simulink model "MSDRPrimaryLoop_LoadFollow"  (R2021b)
settings: Solver=VariableStepAuto  StartTime=0.0  StopTime=604900  MaxStep=1  MinStep=0.01  RelTol=1e-3
undefined symbols (not defined in the file): a_f, A_free_PHX, a_g, A_h_PHX, beta, beta_t, bubbleGeneratorArea, bubbleGeneratorDh, bubbleGeneratorElevation, bubbleGeneratorLength, bubbleGeneratorVolume, bubbleSaturationLevel, bubbleSeparatorArea, bubbleSeparatorDiameter, bubbleSeparatorDo, bubbleSeparatorLength, bubbleSeparatorSlope, bypassRatio, C0, coreFlowArea, coreFuelVolume, coreLowerPlenumArea, coreLowerPlenumHydraulicDiameter, coreLowerPlenumLength, coreLowerPlenumVolume, coreUpperPlenumArea, coreUpperPlenumHydraulicDiameter, coreUpperPlenumLength, coreUpperPlenumVolume, coreVolume, cpGraphite, dissolusionRatio, dMin, dScale, dsmConst, DXeG, Fiss_factor, fuelChannelHydrualicDiameter, fuelChannelLength, fuelDepositRatio, fuelFraction, fuelGraphiteArea, fuelGraphiteHeatTransferCoefficient, gamma0, gamma1, gamma2, generatorDsm, graphiteKDiff, graphiteUnitCellThickness, initialIodineConcentration, InitialXeMolarConcentration, InjectionRatio, injectionRatio, iodineDecayConstant, IodineDecayConstant, iodineYield, kGraphite, kScale, Lam, lam ... (+60)
libraries: fl_lib x268, nesl_utility x106, SimscapeFluids_lib x20, slpidlib x1
(part 7 of 12)

== system MSDRPrimaryLoop_LoadFollow/pipeReactorToPump/XenonCalc/Gas ==
  XeGIn : Inport
  Interphase : Inport  Port=2
  GasRef : Inport  Port=3
  VolumeRate : Inport  Port=4
  Add : Sum  Inputs=+---
  Add1 : Sum  Inputs=+-
  Add2 : Sum
  Constant : Constant
  Gain2 : Gain  Gain=xeDecayConstant
  Gain4 : Gain  Gain=0.5/Area
  LiquidFlowRate : Product
  LiquidVolume : Product  Inputs=*/
  MixtureVolume : Gain  Gain=1/Volume
  PhaseMass : Integrator  LimitOutput=on  LowerSaturationLimit=0
  Subsystem : Subsystem  ReferencedSubsystem=GasToAlpha
  XeGOut : Outport
  GxGas : Outport  Port=2
  wires:
  LiquidFlowRate/1 -> XeGOut/1, Add2/2, Add/3
  Subsystem/1 -> Add1/2
  LiquidVolume/1 -> LiquidFlowRate/2
  Add/1 -> PhaseMass/1
  Constant/1 -> Add1/1
  MixtureVolume/1 -> LiquidVolume/1
  Add1/1 -> LiquidVolume/2
  VolumeRate/1 -> LiquidFlowRate/1
  GasRef/1 -> Subsystem/1
  XeGIn/1 -> Add/1, Add2/1
  Gain2/1 -> Add/4
  PhaseMass/1 -> Gain2/1, MixtureVolume/1
  Gain4/1 -> GxGas/1
  Add2/1 -> Gain4/1
  Interphase/1 -> Add/2

== system MSDRPrimaryLoop_LoadFollow/pipeReactorToPump/XenonCalc/InterphaseTranfser ==
  note: This local to volume isn't strick. Either add an integral or reduce the length of the node if variation is large.
  GxSalt : Inport
  GasRef : Inport  Port=2
  GxGas : Inport  Port=3
  PLoss : Inport  Port=4
  VolumeRate : Inport  Port=5
  Constant : Constant  Value=Dh
  Constitutive : Subsystem
      settings: PortSchema="{\"entries\":[{\"content\":{\"sides\":[{\"content\":{\"connectorIds\":[\"In1\",\"LConn1\",\"In2\",\"In3\",\"In4\"]},\"type\":\"ConnectorPlacement.EquallySpacedRectSide\",\"uuid\":\"b30af6c3-7c55-4661-bc76-939f1c8a4177\"},{\"content\":{\"connectorIds\":[\"Out1\",\"Out2\",\"Out3\",\"Out4\",\"Out5\",\"Out6\",\"Out7\",\"Out8\",\"Out9\"],\"side\":\"RIGHT\"},\"type\":\"ConnectorPlacement.EquallySpacedRectSide\",\"uuid\":\"0b137634-5e01-4bd6-8381-72b0699f5835\"},{\"content\":{\"connectorIds\":[],\"side\":\"TOP\"},\"type\":\"ConnectorPlacement.EquallySpacedRectSide\",\"uuid\":\"06046061-3240-493e-a0a3-282c9541adae\"}]},\"type\":\"ConnectorPlacement.EquallySpacedConnector\",\"uuid\":\"b0591291-fd4b-4355-beaa-e569a19c4b12\"}],\"packageUris\":[\"http://schema.mathworks.com/mf0/Connector/R2020b\"],\"version\":\"1.0\"}"
  MixtureVolume : Gain  Gain=Volume
  String Constant : StringConstant  String="\"upwards\""
  Subsystem : Subsystem  ReferencedSubsystem=kCalculation
      settings: PortSchema="{\"entries\":[{\"content\":{\"sides\":[{\"content\":{\"connectorIds\":[\"In2\",\"In3\",\"In4\",\"In5\",\"In6\",\"In7\",\"In8\",\"In1\"]},\"type\":\"ConnectorPlacement.EquallySpacedRectSide\",\"uuid\":\"002a6616-4b3b-4d3e-9efd-a784f6bbe134\"},{\"content\":{\"connectorIds\":[\"Out1\",\"Out2\"],\"side\":\"RIGHT\"},\"type\":\"ConnectorPlacement.EquallySpacedRectSide\",\"uuid\":\"da6acc14-6515-461b-8149-f4cbf493a4dd\"},{\"content\":{\"connectorIds\":[],\"side\":\"TOP\"},\"type\":\"ConnectorPlacement.EquallySpacedRectSide\",\"uuid\":\"939e49a4-f3cd-4ed3-a7a5-6bbefe0ae08a\"}]},\"type\":\"ConnectorPlacement.EquallySpacedConnector\",\"uuid\":\"8f0c794e-eb76-47c6-abaf-8e07cad1f307\"}],\"packageUris\":[\"http://schema.mathworks.com/mf0/Connector/R2020b\"],\"version\":\"1.0\"}"
  Subsystem1 : Subsystem  ReferencedSubsystem=GasToAlpha
  Transfer Term : MATLAB Function  TreatAsAtomicUnit=on
  Ref : PMIOPort  Side=Left
  TranfserRate : Outport
  wires:
  Transfer Term/1(volRate) -> MixtureVolume/1
  MixtureVolume/1 -> TranfserRate/1
  VolumeRate/1 -> Constitutive/3(VolumeRate)
  GasRef/1 -> Subsystem1/1
  Subsystem1/1 -> Constitutive/1(alpha), Transfer Term/3(alpha)
  Constitutive/1(ul) -> Transfer Term/4(ul)
  Constitutive/2(ug) -> Transfer Term/5(ug)
  Constant/1 -> Subsystem/7, Constitutive/4(Diam)
  GxSalt/1 -> Transfer Term/1(GxS)
  GxGas/1 -> Transfer Term/2(GxG)
  Subsystem/1 -> Transfer Term/7(dsm)
  Subsystem/2 -> Transfer Term/8(k)
  PLoss/1 -> Constitutive/2(PLoss)
  Constitutive/4(Re) -> Subsystem/2
  Constitutive/3(K) -> Transfer Term/6(K)
  Constitutive/5(Sc) -> Subsystem/3
  Constitutive/6(Diff) -> Subsystem/4
  Constitutive/7(alphaC) -> Subsystem/5
  Constitutive/8(dsm) -> Subsystem/6
  Constitutive/9(f_m) -> Subsystem/1
  String Constant/1 -> Subsystem/8
  connections:
  Constitutive/LConn1 -- Ref/RConn1

== system MSDRPrimaryLoop_LoadFollow/pipeReactorToPump/XenonCalc/Salt ==
  XeLIn : Inport  PortDimensions=1
  IodineSNumberDensity : Inport  Port=2  PortDimensions=1
  T_f_ave : Inport  Port=3
  GasRef : Inport  Port=4  PortDimensions=1
  VolumeRate : Inport  Port=5
  Interphase : Inport  Port=6
  Add : Sum  Inputs=+++--  InputSameDT=on
  Add1 : Sum
  Decay : Gain  Gain=xeDecayConstant
  Gain1 : Gain  Gain=0.5/Area
  InPipeGeneration : Subsystem
      settings: PortSchema="{\"entries\":[{\"content\":{\"sides\":[{\"content\":{\"connectorIds\":[\"In1\"]},\"type\":\"ConnectorPlacement.EquallySpacedRectSide\",\"uuid\":\"cf58f9e2-4051-4ec0-bfd5-a375f3464f67\"},{\"content\":{\"connectorIds\":[\"Out1\"],\"side\":\"RIGHT\"},\"type\":\"ConnectorPlacement.EquallySpacedRectSide\",\"uuid\":\"cf475b22-0422-4ebc-b148-ab559744c6ba\"},{\"content\":{\"connectorIds\":[],\"side\":\"TOP\"},\"type\":\"ConnectorPlacement.EquallySpacedRectSide\",\"uuid\":\"15cc78ce-ee79-4f49-b098-b77c0b2a8ba1\"},{\"content\":{\"connectorIds\":[\"In2\"],\"side\":\"BOTTOM\"},\"type\":\"ConnectorPlacement.EquallySpacedRectSide\",\"uuid\":\"64f5be1f-19d6-4b5f-ac24-c41659a6a539\"}]},\"type\":\"ConnectorPlacement.EquallySpacedConnector\",\"uuid\":\"1fb1607a-ceed-4d70-a511-7b706be0d7ea\"}],\"packageUris\":[\"http://schema.mathworks.com/mf0/Connector/R2020b\"],\"version\":\"1.0\"}"
  LiquidFlowRate : Product
  LiquidVolume : Product  Inputs=*/
  MixtureVolume : Gain  Gain=1/Volume
  PhaseMass : Integrator  LimitOutput=on  LowerSaturationLimit=0
  Subsystem1 : Subsystem
  XeLOut : Outport  PortDimensions=1
  GxSalt : Outport  Port=2
  wires:
  LiquidFlowRate/1 -> Add/5, XeLOut/1, Add1/2
  IodineSNumberDensity/1 -> InPipeGeneration/1(IodineSNumberDensity)
  LiquidVolume/1 -> LiquidFlowRate/2
  Add/1 -> PhaseMass/1
  MixtureVolume/1 -> LiquidVolume/1
  VolumeRate/1 -> LiquidFlowRate/1
  T_f_ave/1 -> InPipeGeneration/2(T_f_ave)
  PhaseMass/1 -> Decay/1, MixtureVolume/1
  GasRef/1 -> Subsystem1/1(Gas)
  Subsystem1/1(1-alpha) -> LiquidVolume/2
  InPipeGeneration/1("XenonGenerationRate, [kg/s]") -> Add/2
  XeLIn/1 -> Add1/1, Add/1
  Add1/1 -> Gain1/1
  Gain1/1 -> GxSalt/1
  Interphase/1 -> Add/3
  Decay/1 -> Add/4

== system MSDRPrimaryLoop_LoadFollow/Chemical Processing/Bubble Generator/XenonCalc/Gas ==
  XeGIn : Inport
  Interphase : Inport  Port=2
  GasRef : Inport  Port=3
  VolumeRate : Inport  Port=4
  Add : Sum  Inputs=+---
  Add1 : Sum  Inputs=+-
  Add2 : Sum
  Constant : Constant
  Gain2 : Gain  Gain=xeDecayConstant
  Gain4 : Gain  Gain=0.5/Area
  LiquidFlowRate : Product
  LiquidVolume : Product  Inputs=*/
  MixtureVolume : Gain  Gain=1/Volume
  PhaseMass : Integrator  LimitOutput=on  LowerSaturationLimit=0
  Subsystem : Subsystem  ReferencedSubsystem=GasToAlpha
  XeGOut : Outport
  GxGas : Outport  Port=2
  wires:
  LiquidFlowRate/1 -> XeGOut/1, Add2/2, Add/3
  Subsystem/1 -> Add1/2
  LiquidVolume/1 -> LiquidFlowRate/2
  Add/1 -> PhaseMass/1
  Constant/1 -> Add1/1
  MixtureVolume/1 -> LiquidVolume/1
  Add1/1 -> LiquidVolume/2
  VolumeRate/1 -> LiquidFlowRate/1
  GasRef/1 -> Subsystem/1
  XeGIn/1 -> Add/1, Add2/1
  Gain2/1 -> Add/4
  PhaseMass/1 -> Gain2/1, MixtureVolume/1
  Gain4/1 -> GxGas/1
  Add2/1 -> Gain4/1
  Interphase/1 -> Add/2

== system MSDRPrimaryLoop_LoadFollow/Chemical Processing/Bubble Generator/XenonCalc/InterphaseTranfser ==
  note: This local to volume isn't strick. Either add an integral or reduce the length of the node if variation is large.
  GxSalt : Inport
  GasRef : Inport  Port=2
  GxGas : Inport  Port=3
  PLoss : Inport  Port=4
  VolumeRate : Inport  Port=5
  Constant : Constant  Value=Dh
  Constitutive : Subsystem
      settings: PortSchema="{\"entries\":[{\"content\":{\"sides\":[{\"content\":{\"connectorIds\":[\"In1\",\"LConn1\",\"In2\",\"In3\",\"In4\"]},\"type\":\"ConnectorPlacement.EquallySpacedRectSide\",\"uuid\":\"b30af6c3-7c55-4661-bc76-939f1c8a4177\"},{\"content\":{\"connectorIds\":[\"Out1\",\"Out2\",\"Out3\",\"Out4\",\"Out5\",\"Out6\",\"Out7\",\"Out8\",\"Out9\"],\"side\":\"RIGHT\"},\"type\":\"ConnectorPlacement.EquallySpacedRectSide\",\"uuid\":\"0b137634-5e01-4bd6-8381-72b0699f5835\"},{\"content\":{\"connectorIds\":[],\"side\":\"TOP\"},\"type\":\"ConnectorPlacement.EquallySpacedRectSide\",\"uuid\":\"06046061-3240-493e-a0a3-282c9541adae\"}]},\"type\":\"ConnectorPlacement.EquallySpacedConnector\",\"uuid\":\"b0591291-fd4b-4355-beaa-e569a19c4b12\"}],\"packageUris\":[\"http://schema.mathworks.com/mf0/Connector/R2020b\"],\"version\":\"1.0\"}"
  MixtureVolume : Gain  Gain=Volume
  Subsystem : Subsystem  ReferencedSubsystem=kCalculation
      settings: PortSchema="{\"entries\":[{\"content\":{\"sides\":[{\"content\":{\"connectorIds\":[\"In2\",\"In3\",\"In4\",\"In5\",\"In6\",\"In7\",\"In8\",\"In1\"]},\"type\":\"ConnectorPlacement.EquallySpacedRectSide\",\"uuid\":\"002a6616-4b3b-4d3e-9efd-a784f6bbe134\"},{\"content\":{\"connectorIds\":[\"Out1\",\"Out2\"],\"side\":\"RIGHT\"},\"type\":\"ConnectorPlacement.EquallySpacedRectSide\",\"uuid\":\"da6acc14-6515-461b-8149-f4cbf493a4dd\"},{\"content\":{\"connectorIds\":[],\"side\":\"TOP\"},\"type\":\"ConnectorPlacement.EquallySpacedRectSide\",\"uuid\":\"939e49a4-f3cd-4ed3-a7a5-6bbefe0ae08a\"}]},\"type\":\"ConnectorPlacement.EquallySpacedConnector\",\"uuid\":\"8f0c794e-eb76-47c6-abaf-8e07cad1f307\"}],\"packageUris\":[\"http://schema.mathworks.com/mf0/Connector/R2020b\"],\"version\":\"1.0\"}"
  Subsystem1 : Subsystem  ReferencedSubsystem=GasToAlpha
  Transfer Term : MATLAB Function  TreatAsAtomicUnit=on
  Ref : PMIOPort  Side=Left
  TranfserRate : Outport
  wires:
  Transfer Term/1(volRate) -> MixtureVolume/1
  MixtureVolume/1 -> TranfserRate/1
  VolumeRate/1 -> Constitutive/3(VolumeRate)
  GasRef/1 -> Subsystem1/1
  Subsystem1/1 -> Constitutive/1(alpha), Transfer Term/3(alpha)
  Constitutive/1(ul) -> Transfer Term/4(ul)
  Constitutive/2(ug) -> Transfer Term/5(ug)
  Constant/1 -> Subsystem/7, Constitutive/4(Diam)
  GxSalt/1 -> Transfer Term/1(GxS)
  GxGas/1 -> Transfer Term/2(GxG)
  Subsystem/1 -> Transfer Term/7(dsm)
  Subsystem/2 -> Transfer Term/8(k)
  PLoss/1 -> Constitutive/2(PLoss)
  Constitutive/4(Re) -> Subsystem/2
  Constitutive/3(K) -> Transfer Term/6(K)
  Constitutive/5(Sc) -> Subsystem/3
  Constitutive/6(Diff) -> Subsystem/4
  Constitutive/7(alphaC) -> Subsystem/5
  Constitutive/8(dsm) -> Subsystem/6
  Constitutive/9(f_m) -> Subsystem/1
  connections:
  Constitutive/LConn1 -- Ref/RConn1

== system MSDRPrimaryLoop_LoadFollow/Chemical Processing/Bubble Generator/XenonCalc/Salt ==
  XeLIn : Inport  PortDimensions=1
  IodineSNumberDensity : Inport  Port=2  PortDimensions=1
  T_f_ave : Inport  Port=3
  GasRef : Inport  Port=4  PortDimensions=1
  VolumeRate : Inport  Port=5
  Interphase : Inport  Port=6
  Add : Sum  Inputs=+++--  InputSameDT=on
  Add1 : Sum
  Decay : Gain  Gain=xeDecayConstant
  Gain1 : Gain  Gain=0.5/Area
  InPipeGeneration : Subsystem
      settings: PortSchema="{\"entries\":[{\"content\":{\"sides\":[{\"content\":{\"connectorIds\":[\"In1\"]},\"type\":\"ConnectorPlacement.EquallySpacedRectSide\",\"uuid\":\"cf58f9e2-4051-4ec0-bfd5-a375f3464f67\"},{\"content\":{\"connectorIds\":[\"Out1\"],\"side\":\"RIGHT\"},\"type\":\"ConnectorPlacement.EquallySpacedRectSide\",\"uuid\":\"cf475b22-0422-4ebc-b148-ab559744c6ba\"},{\"content\":{\"connectorIds\":[],\"side\":\"TOP\"},\"type\":\"ConnectorPlacement.EquallySpacedRectSide\",\"uuid\":\"15cc78ce-ee79-4f49-b098-b77c0b2a8ba1\"},{\"content\":{\"connectorIds\":[\"In2\"],\"side\":\"BOTTOM\"},\"type\":\"ConnectorPlacement.EquallySpacedRectSide\",\"uuid\":\"64f5be1f-19d6-4b5f-ac24-c41659a6a539\"}]},\"type\":\"ConnectorPlacement.EquallySpacedConnector\",\"uuid\":\"1fb1607a-ceed-4d70-a511-7b706be0d7ea\"}],\"packageUris\":[\"http://schema.mathworks.com/mf0/Connector/R2020b\"],\"version\":\"1.0\"}"
  LiquidFlowRate : Product
  LiquidVolume : Product  Inputs=*/
  MixtureVolume : Gain  Gain=1/Volume
  PhaseMass : Integrator  LimitOutput=on  LowerSaturationLimit=0
  Subsystem1 : Subsystem
  XeLOut : Outport  PortDimensions=1
  GxSalt : Outport  Port=2
  wires:
  LiquidFlowRate/1 -> Add/5, XeLOut/1, Add1/2
  IodineSNumberDensity/1 -> InPipeGeneration/1(IodineSNumberDensity)
  LiquidVolume/1 -> LiquidFlowRate/2
  Add/1 -> PhaseMass/1
  MixtureVolume/1 -> LiquidVolume/1
  VolumeRate/1 -> LiquidFlowRate/1
  T_f_ave/1 -> InPipeGeneration/2(T_f_ave)
  PhaseMass/1 -> Decay/1, MixtureVolume/1
  GasRef/1 -> Subsystem1/1(Gas)
  Subsystem1/1(1-alpha) -> LiquidVolume/2
  InPipeGeneration/1("XenonGenerationRate, [kg/s]") -> Add/2
  XeLIn/1 -> Add1/1, Add/1
  Add1/1 -> Gain1/1
  Gain1/1 -> GxSalt/1
  Interphase/1 -> Add/3
  Decay/1 -> Add/4

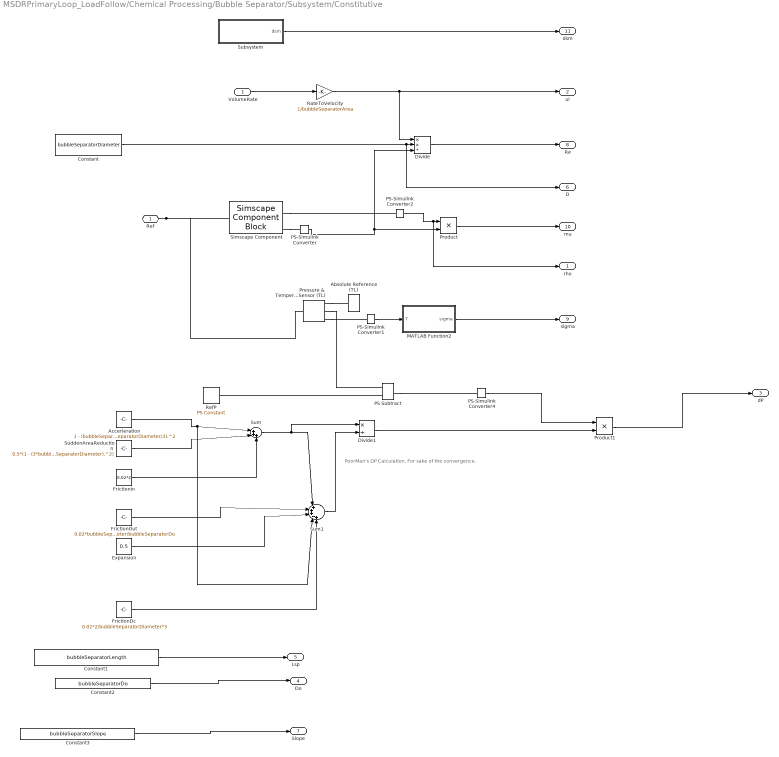
== system MSDRPrimaryLoop_LoadFollow/Chemical Processing/Bubble Separator/Subsystem/Constitutive ==
  note: PoorMan's DP Calculation. For sake of the convergence.
  VolumeRate : Inport
  Absolute Reference (TL) : fl_lib/Thermal Liquid/Elements/Absolute Reference (TL)
      settings: SourceProductBaseCode=SS
  Accerleration : Constant  Value=1 - (bubbleSeparatorDo).^2./(bubbleSeparatorDiameter/3).^2
  Constant : Constant  Value=bubbleSeparatorDiameter
  Constant1 : Constant  Value=bubbleSeparatorLength
  Constant2 : Constant  Value=bubbleSeparatorDo
  Constant3 : Constant  Value=bubbleSeparatorSlope
  Divide : Product  Inputs=**/
  Divide1 : Product  Inputs=*/
  Expansion : Constant  Value=0.5
  FrictionDc : Constant  Value=0.02*2/bubbleSeparatorDiameter*3
  FrictionIn : Constant  Value=0.02*2
  FrictionOut : Constant  Value=0.02*bubbleSeparatorDiameter/bubbleSeparatorDo
  MATLAB Function2 : MATLAB Function  TreatAsAtomicUnit=on
  PS Subtract : fl_lib/Physical Signals/Functions/PS Subtract
  PS-Simulink Converter{,1..2,4} (4 alike) : nesl_utility/PS-Simulink Converter  PhysicalDomain=network_engine_domain  SubClassName=ps_output  LeftPortType=input  RightPortType=output  PseudoPeriodic=off  Frequencies=[]  Unit=inherit  AffineConversion=off
      settings: SourceProductBaseCode=PW,SS
  Pressure & Temperature Sensor (TL) : fl_lib/Thermal Liquid/Sensors/Pressure & Temperature Sensor (TL)
      settings: SourceProductBaseCode=SS  InternalSimscapePortConfiguration="{\"Bottom\":[],\"Left\":[{\"id\":\"A\",\"label\":\"A\",\"type\":\"foundation.thermal_liquid.thermal_liquid\"}],\"Right\":[{\"id\":\"B\",\"label\":\"B\",\"type\":\"foundation.thermal_liquid.thermal_liquid\"},{\"id\":\"P\",\"label\":\"P\",\"type\":\"output\"},{\"id\":\"T\",\"label\":\"T\",\"type\":\"output\"}],\"Top\":[]}"
  Product : Product
  Product1 : Product
  RateToVelocity : Gain  Gain=1/bubbleSeparatorArea
  RefP : fl_lib/Physical Signals/Sources/PS Constant  constant=P0 Pa
  Simscape Component : SimscapeComponentBlock  SourceFile=TL_FullSensor  ComponentPath=TL_FullSensor  ComponentVariants="[\"TL_FullSensor\"]"  ComponentVariantNames="[\"TL_FullSensor\"]"  ClassName=TL_FullSensor  SchemaVersion=1
      settings: CopyFcn=simscape.engine.sli.internal.componentblockcallback(gcbh,'COPY')  PreCopyFcn=simscape.engine.sli.internal.componentblockcallback(gcbh,'PRECOPY')  PreDeleteFcn=simscape.engine.sli.internal.componentblockcallback(gcbh,'PREDELETE')  InternalSimscapePortConfiguration="{\"Bottom\":[],\"Left\":[{\"id\":\"A\",\"label\":\"A\",\"type\":\"foundation.thermal_liquid.thermal_liquid\"}],\"Right\":[{\"id\":\"U\",\"label\":\"u\",\"type\":\"output\"},{\"id\":\"RHO\",\"label\":\"rho\",\"type\":\"output\"},{\"id\":\"CP\",\"label\":\"cp\",\"type\":\"output\"},{\"id\":\"NU\",\"label\":\"nu\",\"type\":\"output\"}],\"Top\":[]}"
      mask Type: Thermodynamic Properties Sensor (TL)
  Subsystem : Subsystem
  SuddenAreaReduction : Constant  Value=0.5*(1 - (3*bubbleSeparatorDo).^2./(bubbleSeparatorDiameter).^2)
  Sum : Sum  Inputs=|+++
  Sum1 : Sum  Inputs=|+++-+
  Ref : PMIOPort  Side=Left
  rho : Outport
  ul : Outport  Port=2
  dP : Outport  Port=3
  Do : Outport  Port=4
  Lsp : Outport  Port=5
  D : Outport  Port=6
  Slope : Outport  Port=7
  Re : Outport  Port=8
  sigma : Outport  Port=9
  mu : Outport  Port=10
  dsm : Outport  Port=11
  wires:
  VolumeRate/1 -> RateToVelocity/1
  RateToVelocity/1 -> ul/1, Divide/1
  PS-Simulink Converter/1 -> Product/2, Divide/3
  Subsystem/1(dsm) -> dsm/1
  Divide/1 -> Re/1
  PS-Simulink Converter1/1 -> MATLAB Function2/1(T)
  MATLAB Function2/1(sigma) -> sigma/1
  PS-Simulink Converter2/1 -> rho/1, Product/1
  Product/1 -> mu/1
  Constant/1 -> D/1, Divide/2
  Product1/1 -> dP/1
  Constant1/1 -> Lsp/1
  Constant2/1 -> Do/1
  Constant3/1 -> Slope/1
  PS-Simulink Converter4/1 -> Product1/1
  Divide1/1 -> Product1/2
  Sum1/1 -> Divide1/2
  Accerleration/1 -> Sum1/4, Sum/1
  SuddenAreaReduction/1 -> Sum/2
  FrictionIn/1 -> Sum/3
  Sum/1 -> Sum1/1, Divide1/1
  FrictionOut/1 -> Sum1/2
  Expansion/1 -> Sum1/3
  FrictionDc/1 -> Sum1/5
  connections:
  Ref/RConn1 -- Pressure & Temperature Sensor (TL)/LConn1 -- Simscape Component/LConn1
  Simscape Component/RConn4 -- PS-Simulink Converter/LConn1
  Pressure & Temperature Sensor (TL)/RConn3 -- PS-Simulink Converter1/LConn1
  Pressure & Temperature Sensor (TL)/RConn1 -- Absolute Reference (TL)/LConn1
  Simscape Component/RConn2 -- PS-Simulink Converter2/LConn1
  Pressure & Temperature Sensor (TL)/RConn2 -- PS Subtract/LConn1
  PS Subtract/LConn2 -- RefP/RConn1
  PS Subtract/RConn1 -- PS-Simulink Converter4/LConn1

== system MSDRPrimaryLoop_LoadFollow/Chemical Processing/ElevationPipe/XenonCalc/Gas ==
  XeGIn : Inport
  Interphase : Inport  Port=2
  GasRef : Inport  Port=3
  VolumeRate : Inport  Port=4
  Add : Sum  Inputs=+---
  Add1 : Sum  Inputs=+-
  Add2 : Sum
  Constant : Constant
  Gain2 : Gain  Gain=xeDecayConstant
  Gain4 : Gain  Gain=0.5/Area
  LiquidFlowRate : Product
  LiquidVolume : Product  Inputs=*/
  MixtureVolume : Gain  Gain=1/Volume
  PhaseMass : Integrator  LimitOutput=on  LowerSaturationLimit=0
  Subsystem : Subsystem  ReferencedSubsystem=GasToAlpha
  XeGOut : Outport
  GxGas : Outport  Port=2
  wires:
  LiquidFlowRate/1 -> XeGOut/1, Add2/2, Add/3
  Subsystem/1 -> Add1/2
  LiquidVolume/1 -> LiquidFlowRate/2
  Add/1 -> PhaseMass/1
  Constant/1 -> Add1/1
  MixtureVolume/1 -> LiquidVolume/1
  Add1/1 -> LiquidVolume/2
  VolumeRate/1 -> LiquidFlowRate/1
  GasRef/1 -> Subsystem/1
  XeGIn/1 -> Add/1, Add2/1
  Gain2/1 -> Add/4
  PhaseMass/1 -> Gain2/1, MixtureVolume/1
  Gain4/1 -> GxGas/1
  Add2/1 -> Gain4/1
  Interphase/1 -> Add/2

== system MSDRPrimaryLoop_LoadFollow/Chemical Processing/ElevationPipe/XenonCalc/InterphaseTranfser1 ==
  GxSalt : Inport
  GasRef : Inport  Port=2
  GxGas : Inport  Port=3
  PLoss : Inport  Port=4
  VolumeRate : Inport  Port=5
  Constant : Constant  Value=Dh
  Constant1 : Constant  Value=Length
  Constant2 : Constant  Value=Area
  Constitutive : Subsystem
      settings: PortSchema="{\"entries\":[{\"content\":{\"sides\":[{\"content\":{\"connectorIds\":[\"In1\",\"LConn1\",\"In2\",\"In3\",\"In4\"]},\"type\":\"ConnectorPlacement.EquallySpacedRectSide\",\"uuid\":\"b30af6c3-7c55-4661-bc76-939f1c8a4177\"},{\"content\":{\"connectorIds\":[\"Out1\",\"Out2\",\"Out3\",\"Out4\",\"Out5\",\"Out6\",\"Out7\",\"Out8\",\"Out9\"],\"side\":\"RIGHT\"},\"type\":\"ConnectorPlacement.EquallySpacedRectSide\",\"uuid\":\"0b137634-5e01-4bd6-8381-72b0699f5835\"},{\"content\":{\"connectorIds\":[],\"side\":\"TOP\"},\"type\":\"ConnectorPlacement.EquallySpacedRectSide\",\"uuid\":\"06046061-3240-493e-a0a3-282c9541adae\"}]},\"type\":\"ConnectorPlacement.EquallySpacedConnector\",\"uuid\":\"b0591291-fd4b-4355-beaa-e569a19c4b12\"}],\"packageUris\":[\"http://schema.mathworks.com/mf0/Connector/R2020b\"],\"version\":\"1.0\"}"
  Long Pipe Averaged Transfer Term : MATLAB Function  TreatAsAtomicUnit=on
  String Constant : StringConstant  String="\"downwards\""
  Subsystem : Subsystem  ReferencedSubsystem=kCalculation
      settings: PortSchema="{\"entries\":[{\"content\":{\"sides\":[{\"content\":{\"connectorIds\":[\"In2\",\"In3\",\"In4\",\"In5\",\"In6\",\"In7\",\"In1\"]},\"type\":\"ConnectorPlacement.EquallySpacedRectSide\",\"uuid\":\"002a6616-4b3b-4d3e-9efd-a784f6bbe134\"},{\"content\":{\"connectorIds\":[\"Out1\",\"Out2\"],\"side\":\"RIGHT\"},\"type\":\"ConnectorPlacement.EquallySpacedRectSide\",\"uuid\":\"da6acc14-6515-461b-8149-f4cbf493a4dd\"},{\"content\":{\"connectorIds\":[],\"side\":\"TOP\"},\"type\":\"ConnectorPlacement.EquallySpacedRectSide\",\"uuid\":\"939e49a4-f3cd-4ed3-a7a5-6bbefe0ae08a\"},{\"content\":{\"connectorIds\":[\"In8\"],\"side\":\"BOTTOM\"},\"type\":\"ConnectorPlacement.EquallySpacedRectSide\",\"uuid\":\"729274ed-8bc2-4a10-a9de-a9d30955ca9f\"}]},\"type\":\"ConnectorPlacement.EquallySpacedConnector\",\"uuid\":\"8f0c794e-eb76-47c6-abaf-8e07cad1f307\"}],\"packageUris\":[\"http://schema.mathworks.com/mf0/Connector/R2020b\"],\"version\":\"1.0\"}"
  Subsystem1 : Subsystem  ReferencedSubsystem=GasToAlpha
  Ref : PMIOPort  Side=Left
  TranfserRate : Outport
  wires:
  Long Pipe Averaged Transfer Term/1(transferRate) -> TranfserRate/1
  VolumeRate/1 -> Constitutive/3(VolumeRate)
  GasRef/1 -> Subsystem1/1
  Subsystem1/1 -> Constitutive/1(alpha), Long Pipe Averaged Transfer Term/3(alpha)
  Constitutive/1(ul) -> Long Pipe Averaged Transfer Term/4(ul)
  Constitutive/2(ug) -> Long Pipe Averaged Transfer Term/5(ug)
  Constant/1 -> Subsystem/7, Constitutive/4(Diam)
  GxSalt/1 -> Long Pipe Averaged Transfer Term/1(GxS)
  GxGas/1 -> Long Pipe Averaged Transfer Term/2(GxG)
  Subsystem/1 -> Long Pipe Averaged Transfer Term/7(dsm)
  Subsystem/2 -> Long Pipe Averaged Transfer Term/8(k)
  PLoss/1 -> Constitutive/2(PLoss)
  Constitutive/4(Re) -> Subsystem/2
  Constitutive/3(K) -> Long Pipe Averaged Transfer Term/6(K)
  Constitutive/5(Sc) -> Subsystem/3
  Constitutive/6(Diff) -> Subsystem/4
  Constitutive/7(alphaC) -> Subsystem/5
  Constitutive/8(dsm) -> Subsystem/6
  Constitutive/9(f_m) -> Subsystem/1
  Constant1/1 -> Long Pipe Averaged Transfer Term/9(L)
  Constant2/1 -> Long Pipe Averaged Transfer Term/10(Area)
  String Constant/1 -> Subsystem/8
  connections:
  Constitutive/LConn1 -- Ref/RConn1

== system MSDRPrimaryLoop_LoadFollow/Chemical Processing/ElevationPipe/XenonCalc/Salt ==
  XeLIn : Inport  PortDimensions=1
  IodineSNumberDensity : Inport  Port=2  PortDimensions=1
  T_f_ave : Inport  Port=3
  GasRef : Inport  Port=4  PortDimensions=1
  VolumeRate : Inport  Port=5
  Interphase : Inport  Port=6
  Add : Sum  Inputs=+++--  InputSameDT=on
  Decay : Gain  Gain=xeDecayConstant
  Gain1 : Gain  Gain=1/Area
  InPipeGeneration : Subsystem
      settings: PortSchema="{\"entries\":[{\"content\":{\"sides\":[{\"content\":{\"connectorIds\":[\"In1\"]},\"type\":\"ConnectorPlacement.EquallySpacedRectSide\",\"uuid\":\"cf58f9e2-4051-4ec0-bfd5-a375f3464f67\"},{\"content\":{\"connectorIds\":[\"Out1\"],\"side\":\"RIGHT\"},\"type\":\"ConnectorPlacement.EquallySpacedRectSide\",\"uuid\":\"cf475b22-0422-4ebc-b148-ab559744c6ba\"},{\"content\":{\"connectorIds\":[],\"side\":\"TOP\"},\"type\":\"ConnectorPlacement.EquallySpacedRectSide\",\"uuid\":\"15cc78ce-ee79-4f49-b098-b77c0b2a8ba1\"},{\"content\":{\"connectorIds\":[\"In2\"],\"side\":\"BOTTOM\"},\"type\":\"ConnectorPlacement.EquallySpacedRectSide\",\"uuid\":\"64f5be1f-19d6-4b5f-ac24-c41659a6a539\"}]},\"type\":\"ConnectorPlacement.EquallySpacedConnector\",\"uuid\":\"1fb1607a-ceed-4d70-a511-7b706be0d7ea\"}],\"packageUris\":[\"http://schema.mathworks.com/mf0/Connector/R2020b\"],\"version\":\"1.0\"}"
  LiquidFlowRate : Product
  LiquidVolume : Product  Inputs=*/
  MixtureVolume : Gain  Gain=1/Volume
  PhaseMass : Integrator  LimitOutput=on  LowerSaturationLimit=0
  Subsystem1 : Subsystem
  XeLOut : Outport  PortDimensions=1
  GxSalt : Outport  Port=2
  wires:
  LiquidFlowRate/1 -> Add/5, XeLOut/1
  IodineSNumberDensity/1 -> InPipeGeneration/1(IodineSNumberDensity)
  LiquidVolume/1 -> LiquidFlowRate/2
  Add/1 -> PhaseMass/1
  MixtureVolume/1 -> LiquidVolume/1
  VolumeRate/1 -> LiquidFlowRate/1
  T_f_ave/1 -> InPipeGeneration/2(T_f_ave)
  PhaseMass/1 -> Decay/1, MixtureVolume/1
  GasRef/1 -> Subsystem1/1(Gas)
  Subsystem1/1(1-alpha) -> LiquidVolume/2
  InPipeGeneration/1("XenonGenerationRate, [kg/s]") -> Add/2
  XeLIn/1 -> Gain1/1, Add/1
  Gain1/1 -> GxSalt/1
  Interphase/1 -> Add/3
  Decay/1 -> Add/4

== system MSDRPrimaryLoop_LoadFollow/Chemical Processing/PipeLine/XenonCalc/Gas ==
  XeGIn : Inport
  Interphase : Inport  Port=2
  GasRef : Inport  Port=3
  VolumeRate : Inport  Port=4
  Add : Sum  Inputs=+---
  Add1 : Sum  Inputs=+-
  Add2 : Sum
  Constant : Constant
  Gain2 : Gain  Gain=xeDecayConstant
  Gain4 : Gain  Gain=0.5/Area
  LiquidFlowRate : Product
  LiquidVolume : Product  Inputs=*/
  MixtureVolume : Gain  Gain=1/Volume
  PhaseMass : Integrator  LimitOutput=on  LowerSaturationLimit=0
  Subsystem : Subsystem  ReferencedSubsystem=GasToAlpha
  XeGOut : Outport
  GxGas : Outport  Port=2
  wires:
  LiquidFlowRate/1 -> XeGOut/1, Add2/2, Add/3
  Subsystem/1 -> Add1/2
  LiquidVolume/1 -> LiquidFlowRate/2
  Add/1 -> PhaseMass/1
  Constant/1 -> Add1/1
  MixtureVolume/1 -> LiquidVolume/1
  Add1/1 -> LiquidVolume/2
  VolumeRate/1 -> LiquidFlowRate/1
  GasRef/1 -> Subsystem/1
  XeGIn/1 -> Add/1, Add2/1
  Gain2/1 -> Add/4
  PhaseMass/1 -> Gain2/1, MixtureVolume/1
  Gain4/1 -> GxGas/1
  Add2/1 -> Gain4/1
  Interphase/1 -> Add/2

== system MSDRPrimaryLoop_LoadFollow/Chemical Processing/PipeLine/XenonCalc/InterphaseTranfser ==
  GxSalt : Inport
  GasRef : Inport  Port=2
  GxGas : Inport  Port=3
  PLoss : Inport  Port=4
  VolumeRate : Inport  Port=5
  Constant : Constant  Value=Dh
  Constant1 : Constant  Value=Length
  Constant2 : Constant  Value=Area
  Constant3 : Constant  Value=0.5
  Constitutive : Subsystem
      settings: PortSchema="{\"entries\":[{\"content\":{\"sides\":[{\"content\":{\"connectorIds\":[\"In1\",\"LConn1\",\"In2\",\"In3\",\"In4\"]},\"type\":\"ConnectorPlacement.EquallySpacedRectSide\",\"uuid\":\"b30af6c3-7c55-4661-bc76-939f1c8a4177\"},{\"content\":{\"connectorIds\":[\"Out1\",\"Out2\",\"Out3\",\"Out4\",\"Out5\",\"Out6\",\"Out7\",\"Out8\",\"Out9\"],\"side\":\"RIGHT\"},\"type\":\"ConnectorPlacement.EquallySpacedRectSide\",\"uuid\":\"0b137634-5e01-4bd6-8381-72b0699f5835\"},{\"content\":{\"connectorIds\":[],\"side\":\"TOP\"},\"type\":\"ConnectorPlacement.EquallySpacedRectSide\",\"uuid\":\"06046061-3240-493e-a0a3-282c9541adae\"}]},\"type\":\"ConnectorPlacement.EquallySpacedConnector\",\"uuid\":\"b0591291-fd4b-4355-beaa-e569a19c4b12\"}],\"packageUris\":[\"http://schema.mathworks.com/mf0/Connector/R2020b\"],\"version\":\"1.0\"}"
  Long Pipe Averaged Transfer Term : MATLAB Function  TreatAsAtomicUnit=on
  Subsystem : Subsystem  ReferencedSubsystem=kCalculation
      settings: PortSchema="{\"entries\":[{\"content\":{\"sides\":[{\"content\":{\"connectorIds\":[\"In2\",\"In3\",\"In4\",\"In5\",\"In6\",\"In7\",\"In8\",\"In1\"]},\"type\":\"ConnectorPlacement.EquallySpacedRectSide\",\"uuid\":\"002a6616-4b3b-4d3e-9efd-a784f6bbe134\"},{\"content\":{\"connectorIds\":[\"Out1\",\"Out2\"],\"side\":\"RIGHT\"},\"type\":\"ConnectorPlacement.EquallySpacedRectSide\",\"uuid\":\"da6acc14-6515-461b-8149-f4cbf493a4dd\"},{\"content\":{\"connectorIds\":[],\"side\":\"TOP\"},\"type\":\"ConnectorPlacement.EquallySpacedRectSide\",\"uuid\":\"939e49a4-f3cd-4ed3-a7a5-6bbefe0ae08a\"}]},\"type\":\"ConnectorPlacement.EquallySpacedConnector\",\"uuid\":\"8f0c794e-eb76-47c6-abaf-8e07cad1f307\"}],\"packageUris\":[\"http://schema.mathworks.com/mf0/Connector/R2020b\"],\"version\":\"1.0\"}"
  Subsystem1 : Subsystem  ReferencedSubsystem=GasToAlpha
  Ref : PMIOPort  Side=Left
  TranfserRate : Outport
  wires:
  Long Pipe Averaged Transfer Term/1(transferRate) -> TranfserRate/1
  VolumeRate/1 -> Constitutive/3(VolumeRate)
  GasRef/1 -> Subsystem1/1
  Subsystem1/1 -> Constitutive/1(alpha), Long Pipe Averaged Transfer Term/3(alpha)
  Constitutive/1(ul) -> Long Pipe Averaged Transfer Term/4(ul)
  Constitutive/2(ug) -> Long Pipe Averaged Transfer Term/5(ug)
  Constant/1 -> Subsystem/7, Constitutive/4(Diam)
  GxSalt/1 -> Long Pipe Averaged Transfer Term/1(GxS)
  GxGas/1 -> Long Pipe Averaged Transfer Term/2(GxG)
  Subsystem/1 -> Long Pipe Averaged Transfer Term/7(dsm)
  Subsystem/2 -> Long Pipe Averaged Transfer Term/8(k)
  PLoss/1 -> Constitutive/2(PLoss)
  Constitutive/4(Re) -> Subsystem/2
  Constitutive/3(K) -> Long Pipe Averaged Transfer Term/6(K)
  Constitutive/5(Sc) -> Subsystem/3
  Constitutive/6(Diff) -> Subsystem/4
  Constitutive/7(alphaC) -> Subsystem/5
  Constitutive/8(dsm) -> Subsystem/6
  Constitutive/9(f_m) -> Subsystem/1
  Constant1/1 -> Long Pipe Averaged Transfer Term/9(L)
  Constant2/1 -> Long Pipe Averaged Transfer Term/10(Area)
  Constant3/1 -> Subsystem/8
  connections:
  Constitutive/LConn1 -- Ref/RConn1

== system MSDRPrimaryLoop_LoadFollow/Chemical Processing/PipeLine/XenonCalc/Salt ==
  XeLIn : Inport  PortDimensions=1
  IodineSNumberDensity : Inport  Port=2  PortDimensions=1
  T_f_ave : Inport  Port=3
  GasRef : Inport  Port=4  PortDimensions=1
  VolumeRate : Inport  Port=5
  Interphase : Inport  Port=6
  Add : Sum  Inputs=+++--  InputSameDT=on
  Decay : Gain  Gain=xeDecayConstant
  Gain1 : Gain  Gain=1/Area
  InPipeGeneration : Subsystem
      settings: PortSchema="{\"entries\":[{\"content\":{\"sides\":[{\"content\":{\"connectorIds\":[\"In1\"]},\"type\":\"ConnectorPlacement.EquallySpacedRectSide\",\"uuid\":\"cf58f9e2-4051-4ec0-bfd5-a375f3464f67\"},{\"content\":{\"connectorIds\":[\"Out1\"],\"side\":\"RIGHT\"},\"type\":\"ConnectorPlacement.EquallySpacedRectSide\",\"uuid\":\"cf475b22-0422-4ebc-b148-ab559744c6ba\"},{\"content\":{\"connectorIds\":[],\"side\":\"TOP\"},\"type\":\"ConnectorPlacement.EquallySpacedRectSide\",\"uuid\":\"15cc78ce-ee79-4f49-b098-b77c0b2a8ba1\"},{\"content\":{\"connectorIds\":[\"In2\"],\"side\":\"BOTTOM\"},\"type\":\"ConnectorPlacement.EquallySpacedRectSide\",\"uuid\":\"64f5be1f-19d6-4b5f-ac24-c41659a6a539\"}]},\"type\":\"ConnectorPlacement.EquallySpacedConnector\",\"uuid\":\"1fb1607a-ceed-4d70-a511-7b706be0d7ea\"}],\"packageUris\":[\"http://schema.mathworks.com/mf0/Connector/R2020b\"],\"version\":\"1.0\"}"
  LiquidFlowRate : Product
  LiquidVolume : Product  Inputs=*/
  MixtureVolume : Gain  Gain=1/Volume
  PhaseMass : Integrator  LimitOutput=on  LowerSaturationLimit=0
  Subsystem1 : Subsystem
  XeLOut : Outport  PortDimensions=1
  GxSalt : Outport  Port=2
  wires:
  LiquidFlowRate/1 -> Add/5, XeLOut/1
  IodineSNumberDensity/1 -> InPipeGeneration/1(IodineSNumberDensity)
  LiquidVolume/1 -> LiquidFlowRate/2
  Add/1 -> PhaseMass/1
  MixtureVolume/1 -> LiquidVolume/1
  VolumeRate/1 -> LiquidFlowRate/1
  T_f_ave/1 -> InPipeGeneration/2(T_f_ave)
  PhaseMass/1 -> Decay/1, MixtureVolume/1
  GasRef/1 -> Subsystem1/1(Gas)
  Subsystem1/1(1-alpha) -> LiquidVolume/2
  InPipeGeneration/1("XenonGenerationRate, [kg/s]") -> Add/2
  XeLIn/1 -> Gain1/1, Add/1
  Gain1/1 -> GxSalt/1
  Interphase/1 -> Add/3
  Decay/1 -> Add/4

== system MSDRPrimaryLoop_LoadFollow/PHX/PHX Ideal/PHXIdeal/DP_Ideal ==
  Design Pressure Drop : fl_lib/Physical Signals/Sources/PS Constant  constant=-dP Pa
  DesignFlowRate : fl_lib/Physical Signals/Sources/PS Constant  constant=VDot m^3/s
  Ideal Pressure Drop : fl_lib/Physical Signals/Functions/PS Product
  PS Divide : fl_lib/Physical Signals/Functions/PS Divide
      settings: SourceProductBaseCode=SS
  PS Math Function : fl_lib/Physical Signals/Functions/PS Math Function  fcn_choice=foundation.enum.math_function.square  v=1
      settings: SourceProductBaseCode=SS
  Inlet : PMIOPort  Side=Left
  Outlet : PMIOPort  Port=2  Side=Right
  DP : PMIOPort  Port=3  Side=Right
  VolumeRate : PMIOPort  Port=4  Side=Left
  connections:
  Inlet/RConn1 -- Outlet/RConn1
  Ideal Pressure Drop/RConn1 -- DP/RConn1
  VolumeRate/RConn1 -- PS Divide/LConn1
  DesignFlowRate/RConn1 -- PS Divide/LConn2
  PS Divide/RConn1 -- PS Math Function/LConn1
  Ideal Pressure Drop/LConn1 -- PS Math Function/RConn1
  Ideal Pressure Drop/LConn2 -- Design Pressure Drop/RConn1

== system MSDRPrimaryLoop_LoadFollow/PHX/PHX Ideal/XenonCalc/Gas ==
  XeGIn : Inport
  Interphase : Inport  Port=2
  GasRef : Inport  Port=3
  VolumeRate : Inport  Port=4
  Add : Sum  Inputs=+---
  Add1 : Sum  Inputs=+-
  Add2 : Sum
  Constant : Constant
  Gain2 : Gain  Gain=xeDecayConstant
  Gain4 : Gain  Gain=0.5/Area
  LiquidFlowRate : Product
  LiquidVolume : Product  Inputs=*/
  MixtureVolume : Gain  Gain=1/Volume
  PhaseMass : Integrator  LimitOutput=on  LowerSaturationLimit=0
  Subsystem : Subsystem  ReferencedSubsystem=GasToAlpha
  XeGOut : Outport
  GxGas : Outport  Port=2
  wires:
  LiquidFlowRate/1 -> XeGOut/1, Add2/2, Add/3
  Subsystem/1 -> Add1/2
  LiquidVolume/1 -> LiquidFlowRate/2
  Add/1 -> PhaseMass/1
  Constant/1 -> Add1/1
  MixtureVolume/1 -> LiquidVolume/1
  Add1/1 -> LiquidVolume/2
  VolumeRate/1 -> LiquidFlowRate/1
  GasRef/1 -> Subsystem/1
  XeGIn/1 -> Add/1, Add2/1
  Gain2/1 -> Add/4
  PhaseMass/1 -> Gain2/1, MixtureVolume/1
  Gain4/1 -> GxGas/1
  Add2/1 -> Gain4/1
  Interphase/1 -> Add/2

== system MSDRPrimaryLoop_LoadFollow/PHX/PHX Ideal/XenonCalc/InterphaseTranfser ==
  note: This local to volume isn't strick. Either add an integral or reduce the length of the node if variation is large.
  GxSalt : Inport
  GasRef : Inport  Port=2
  GxGas : Inport  Port=3
  PLoss : Inport  Port=4
  VolumeRate : Inport  Port=5
  Constant : Constant  Value=Dh
  Constant1 : Constant  Value=0.5
  Constitutive : Subsystem
      settings: PortSchema="{\"entries\":[{\"content\":{\"sides\":[{\"content\":{\"connectorIds\":[\"In1\",\"LConn1\",\"In2\",\"In3\",\"In4\"]},\"type\":\"ConnectorPlacement.EquallySpacedRectSide\",\"uuid\":\"b30af6c3-7c55-4661-bc76-939f1c8a4177\"},{\"content\":{\"connectorIds\":[\"Out1\",\"Out2\",\"Out3\",\"Out4\",\"Out5\",\"Out6\",\"Out7\",\"Out8\",\"Out9\"],\"side\":\"RIGHT\"},\"type\":\"ConnectorPlacement.EquallySpacedRectSide\",\"uuid\":\"0b137634-5e01-4bd6-8381-72b0699f5835\"},{\"content\":{\"connectorIds\":[],\"side\":\"TOP\"},\"type\":\"ConnectorPlacement.EquallySpacedRectSide\",\"uuid\":\"06046061-3240-493e-a0a3-282c9541adae\"}]},\"type\":\"ConnectorPlacement.EquallySpacedConnector\",\"uuid\":\"b0591291-fd4b-4355-beaa-e569a19c4b12\"}],\"packageUris\":[\"http://schema.mathworks.com/mf0/Connector/R2020b\"],\"version\":\"1.0\"}"
  MixtureVolume : Gain  Gain=Volume
  Subsystem : Subsystem  ReferencedSubsystem=kCalculation
      settings: PortSchema="{\"entries\":[{\"content\":{\"sides\":[{\"content\":{\"connectorIds\":[\"In2\",\"In3\",\"In4\",\"In5\",\"In6\",\"In7\",\"In8\",\"In1\"]},\"type\":\"ConnectorPlacement.EquallySpacedRectSide\",\"uuid\":\"002a6616-4b3b-4d3e-9efd-a784f6bbe134\"},{\"content\":{\"connectorIds\":[\"Out1\",\"Out2\"],\"side\":\"RIGHT\"},\"type\":\"ConnectorPlacement.EquallySpacedRectSide\",\"uuid\":\"da6acc14-6515-461b-8149-f4cbf493a4dd\"},{\"content\":{\"connectorIds\":[],\"side\":\"TOP\"},\"type\":\"ConnectorPlacement.EquallySpacedRectSide\",\"uuid\":\"939e49a4-f3cd-4ed3-a7a5-6bbefe0ae08a\"}]},\"type\":\"ConnectorPlacement.EquallySpacedConnector\",\"uuid\":\"8f0c794e-eb76-47c6-abaf-8e07cad1f307\"}],\"packageUris\":[\"http://schema.mathworks.com/mf0/Connector/R2020b\"],\"version\":\"1.0\"}"
  Subsystem1 : Subsystem  ReferencedSubsystem=GasToAlpha
  Transfer Term : MATLAB Function  TreatAsAtomicUnit=on
  Ref : PMIOPort  Side=Left
  TranfserRate : Outport
  wires:
  Transfer Term/1(volRate) -> MixtureVolume/1
  MixtureVolume/1 -> TranfserRate/1
  VolumeRate/1 -> Constitutive/3(VolumeRate)
  GasRef/1 -> Subsystem1/1
  Subsystem1/1 -> Constitutive/1(alpha), Transfer Term/3(alpha)
  Constitutive/1(ul) -> Transfer Term/4(ul)
  Constitutive/2(ug) -> Transfer Term/5(ug)
  Constant/1 -> Subsystem/7, Constitutive/4(Diam)
  GxSalt/1 -> Transfer Term/1(GxS)
  GxGas/1 -> Transfer Term/2(GxG)
  Subsystem/1 -> Transfer Term/7(dsm)
  Subsystem/2 -> Transfer Term/8(k)
  PLoss/1 -> Constitutive/2(PLoss)
  Constitutive/4(Re) -> Subsystem/2
  Constitutive/3(K) -> Transfer Term/6(K)
  Constitutive/5(Sc) -> Subsystem/3
  Constitutive/6(Diff) -> Subsystem/4
  Constitutive/7(alphaC) -> Subsystem/5
  Constitutive/8(dsm) -> Subsystem/6
  Constitutive/9(f_m) -> Subsystem/1
  Constant1/1 -> Subsystem/8
  connections:
  Constitutive/LConn1 -- Ref/RConn1

== system MSDRPrimaryLoop_LoadFollow/PHX/PHX Ideal/XenonCalc/Salt ==
  XeLIn : Inport  PortDimensions=1
  IodineSNumberDensity : Inport  Port=2  PortDimensions=1
  T_f_ave : Inport  Port=3
  GasRef : Inport  Port=4  PortDimensions=1
  VolumeRate : Inport  Port=5
  Interphase : Inport  Port=6
  Add : Sum  Inputs=+++--  InputSameDT=on
  Add1 : Sum
  Decay : Gain  Gain=xeDecayConstant
  Gain1 : Gain  Gain=0.5/Area
  InPipeGeneration : Subsystem
      settings: PortSchema="{\"entries\":[{\"content\":{\"sides\":[{\"content\":{\"connectorIds\":[\"In1\"]},\"type\":\"ConnectorPlacement.EquallySpacedRectSide\",\"uuid\":\"cf58f9e2-4051-4ec0-bfd5-a375f3464f67\"},{\"content\":{\"connectorIds\":[\"Out1\"],\"side\":\"RIGHT\"},\"type\":\"ConnectorPlacement.EquallySpacedRectSide\",\"uuid\":\"cf475b22-0422-4ebc-b148-ab559744c6ba\"},{\"content\":{\"connectorIds\":[],\"side\":\"TOP\"},\"type\":\"ConnectorPlacement.EquallySpacedRectSide\",\"uuid\":\"15cc78ce-ee79-4f49-b098-b77c0b2a8ba1\"},{\"content\":{\"connectorIds\":[\"In2\"],\"side\":\"BOTTOM\"},\"type\":\"ConnectorPlacement.EquallySpacedRectSide\",\"uuid\":\"64f5be1f-19d6-4b5f-ac24-c41659a6a539\"}]},\"type\":\"ConnectorPlacement.EquallySpacedConnector\",\"uuid\":\"1fb1607a-ceed-4d70-a511-7b706be0d7ea\"}],\"packageUris\":[\"http://schema.mathworks.com/mf0/Connector/R2020b\"],\"version\":\"1.0\"}"
  LiquidFlowRate : Product
  LiquidVolume : Product  Inputs=*/
  MixtureVolume : Gain  Gain=1/Volume
  PhaseMass : Integrator  LimitOutput=on  LowerSaturationLimit=0
  Subsystem1 : Subsystem
  XeLOut : Outport  PortDimensions=1
  GxSalt : Outport  Port=2
  wires:
  LiquidFlowRate/1 -> Add/5, XeLOut/1, Add1/2
  IodineSNumberDensity/1 -> InPipeGeneration/1(IodineSNumberDensity)
  LiquidVolume/1 -> LiquidFlowRate/2
  Add/1 -> PhaseMass/1
  MixtureVolume/1 -> LiquidVolume/1
  VolumeRate/1 -> LiquidFlowRate/1
  T_f_ave/1 -> InPipeGeneration/2(T_f_ave)
  PhaseMass/1 -> Decay/1, MixtureVolume/1
  GasRef/1 -> Subsystem1/1(Gas)
  Subsystem1/1(1-alpha) -> LiquidVolume/2
  InPipeGeneration/1("XenonGenerationRate, [kg/s]") -> Add/2
  XeLIn/1 -> Add1/1, Add/1
  Add1/1 -> Gain1/1
  Gain1/1 -> GxSalt/1
  Interphase/1 -> Add/3
  Decay/1 -> Add/4

== system MSDRPrimaryLoop_LoadFollow/PHX/PHX Physical/XenonCalc1/Gas ==
  XeGIn : Inport
  Interphase : Inport  Port=2
  GasRef : Inport  Port=3
  VolumeRate : Inport  Port=4
  Add : Sum  Inputs=+---
  Add1 : Sum  Inputs=+-
  Add2 : Sum
  Constant : Constant
  Gain2 : Gain  Gain=XeDecayConstant
  Gain4 : Gain  Gain=0.5/PipeArea
  LiquidFlowRate : Product
  LiquidVolume : Product  Inputs=*/
  MixtureVolume : Gain  Gain=1/PipeVolume
  PhaseMass : Integrator  LimitOutput=on  LowerSaturationLimit=0
  Subsystem : Subsystem  ReferencedSubsystem=GasToAlpha
  XeGOut : Outport
  GxGas : Outport  Port=2
  wires:
  LiquidFlowRate/1 -> XeGOut/1, Add2/2, Add/3
  Subsystem/1 -> Add1/2
  LiquidVolume/1 -> LiquidFlowRate/2
  Add/1 -> PhaseMass/1
  Constant/1 -> Add1/1
  MixtureVolume/1 -> LiquidVolume/1
  Add1/1 -> LiquidVolume/2
  VolumeRate/1 -> LiquidFlowRate/1
  GasRef/1 -> Subsystem/1
  XeGIn/1 -> Add/1, Add2/1
  Gain2/1 -> Add/4
  PhaseMass/1 -> Gain2/1, MixtureVolume/1
  Gain4/1 -> GxGas/1
  Add2/1 -> Gain4/1
  Interphase/1 -> Add/2

== system MSDRPrimaryLoop_LoadFollow/PHX/PHX Physical/XenonCalc1/InterphaseTranfser ==
  note: This local to volume isn't strick. Either add an integral or reduce the length of the node if variation is large.
  GxSalt : Inport
  GasRef : Inport  Port=2
  GxGas : Inport  Port=3
  VolumeRate : Inport  Port=4
  Constant : Constant  Value=Dh
  Constitutive : Subsystem
      settings: PortSchema="{\"entries\":[{\"content\":{\"sides\":[{\"content\":{\"connectorIds\":[\"In1\",\"LConn1\",\"In2\",\"In3\"]},\"type\":\"ConnectorPlacement.EquallySpacedRectSide\",\"uuid\":\"b30af6c3-7c55-4661-bc76-939f1c8a4177\"},{\"content\":{\"connectorIds\":[\"Out1\",\"Out2\",\"Out3\",\"Out4\",\"Out5\",\"Out6\",\"Out7\",\"Out8\"],\"side\":\"RIGHT\"},\"type\":\"ConnectorPlacement.EquallySpacedRectSide\",\"uuid\":\"0b137634-5e01-4bd6-8381-72b0699f5835\"},{\"content\":{\"connectorIds\":[],\"side\":\"TOP\"},\"type\":\"ConnectorPlacement.EquallySpacedRectSide\",\"uuid\":\"06046061-3240-493e-a0a3-282c9541adae\"}]},\"type\":\"ConnectorPlacement.EquallySpacedConnector\",\"uuid\":\"b0591291-fd4b-4355-beaa-e569a19c4b12\"}],\"packageUris\":[\"http://schema.mathworks.com/mf0/Connector/R2020b\"],\"version\":\"1.0\"}"
  MixtureVolume : Gain  Gain=PipeVolume
  Subsystem1 : Subsystem  ReferencedSubsystem=GasToAlpha
  Transfer Term : MATLAB Function  TreatAsAtomicUnit=on
  k Calculation : MATLAB Function  TreatAsAtomicUnit=on
  Ref : PMIOPort  Side=Left
  TranfserRate : Outport
  wires:
  Transfer Term/1(volRate) -> MixtureVolume/1
  MixtureVolume/1 -> TranfserRate/1
  k Calculation/2(k) -> Transfer Term/8(k)
  k Calculation/1(dsm) -> Transfer Term/7(dsm)
  VolumeRate/1 -> Constitutive/2(VolumeRate)
  GasRef/1 -> Subsystem1/1
  Subsystem1/1 -> Constitutive/1(alpha), Transfer Term/3(alpha)
  Constitutive/1(ul) -> Transfer Term/4(ul)
  Constitutive/2(ug) -> Transfer Term/5(ug)
  Constitutive/3(K) -> Transfer Term/6(K)
  Constitutive/4(Re) -> k Calculation/1(Re)
  Constitutive/5(Sc) -> k Calculation/2(Sc)
  Constitutive/6(Diff) -> k Calculation/3(Diff)
  Constitutive/8(dsm) -> k Calculation/5("dsm ")
  Constant/1 -> Constitutive/3(Diam), k Calculation/6(Diam)
  Constitutive/7(alphaC) -> k Calculation/4(alpha)
  GxSalt/1 -> Transfer Term/1(GxS)
  GxGas/1 -> Transfer Term/2(GxG)
  connections:
  Constitutive/LConn1 -- Ref/RConn1

== system MSDRPrimaryLoop_LoadFollow/PHX/PHX Physical/XenonCalc1/Salt ==
  XeLIn : Inport  PortDimensions=1
  IodineSNumberDensity : Inport  Port=2  PortDimensions=1
  T_f_ave : Inport  Port=3
  GasRef : Inport  Port=4  PortDimensions=1
  VolumeRate : Inport  Port=5
  Interphase : Inport  Port=6
  Add : Sum  Inputs=+++--  InputSameDT=on
  Add1 : Sum
  Decay : Gain  Gain=XeDecayConstant
  Gain1 : Gain  Gain=0.5/PipeArea
  InPipeGeneration : Subsystem
      settings: PortSchema="{\"entries\":[{\"content\":{\"sides\":[{\"content\":{\"connectorIds\":[\"In1\"]},\"type\":\"ConnectorPlacement.EquallySpacedRectSide\",\"uuid\":\"cf58f9e2-4051-4ec0-bfd5-a375f3464f67\"},{\"content\":{\"connectorIds\":[\"Out1\"],\"side\":\"RIGHT\"},\"type\":\"ConnectorPlacement.EquallySpacedRectSide\",\"uuid\":\"cf475b22-0422-4ebc-b148-ab559744c6ba\"},{\"content\":{\"connectorIds\":[],\"side\":\"TOP\"},\"type\":\"ConnectorPlacement.EquallySpacedRectSide\",\"uuid\":\"15cc78ce-ee79-4f49-b098-b77c0b2a8ba1\"},{\"content\":{\"connectorIds\":[\"In2\"],\"side\":\"BOTTOM\"},\"type\":\"ConnectorPlacement.EquallySpacedRectSide\",\"uuid\":\"64f5be1f-19d6-4b5f-ac24-c41659a6a539\"}]},\"type\":\"ConnectorPlacement.EquallySpacedConnector\",\"uuid\":\"1fb1607a-ceed-4d70-a511-7b706be0d7ea\"}],\"packageUris\":[\"http://schema.mathworks.com/mf0/Connector/R2020b\"],\"version\":\"1.0\"}"
  LiquidFlowRate : Product
  LiquidVolume : Product  Inputs=*/
  MixtureVolume : Gain  Gain=1/PipeVolume
  PhaseMass : Integrator  InitialCondition=5e-5*PipeVolume  LimitOutput=on  LowerSaturationLimit=0
  Subsystem1 : Subsystem
  XeLOut : Outport  PortDimensions=1
  GxSalt : Outport  Port=2
  wires:
  LiquidFlowRate/1 -> Add/5, XeLOut/1, Add1/2
  IodineSNumberDensity/1 -> InPipeGeneration/1(IodineSNumberDensity)
  LiquidVolume/1 -> LiquidFlowRate/2
  Add/1 -> PhaseMass/1
  MixtureVolume/1 -> LiquidVolume/1
  VolumeRate/1 -> LiquidFlowRate/1
  T_f_ave/1 -> InPipeGeneration/2(T_f_ave)
  PhaseMass/1 -> Decay/1, MixtureVolume/1
  GasRef/1 -> Subsystem1/1(Gas)
  Subsystem1/1(1-alpha) -> LiquidVolume/2
  InPipeGeneration/1("XenonGenerationRate, [kg/s]") -> Add/2
  XeLIn/1 -> Add1/1, Add/1
  Add1/1 -> Gain1/1
  Gain1/1 -> GxSalt/1
  Interphase/1 -> Add/3
  Decay/1 -> Add/4

== system MSDRPrimaryLoop_LoadFollow/Pump/PumpIdeal/XenonCalcPump/Gas ==
  XeGIn : Inport
  Interphase : Inport  Port=2
  GasRef : Inport  Port=3
  VolumeRate : Inport  Port=4
  Add : Sum  Inputs=+---
  Add1 : Sum  Inputs=+-
  Constant : Constant
  Constant1 : Constant  Value=0.001
  Divide : Product  Inputs=*/
  Gain2 : Gain  Gain=xeDecayConstant
  LiquidFlowRate : Product
  LiquidVolume : Product  Inputs=*/
  MixtureVolume : Gain  Gain=1/PipeVolume
  PhaseMass : Integrator  LimitOutput=on  LowerSaturationLimit=0
  PreventDivideByZero : MinMax  Function=max  Inputs=2
  Subsystem : Subsystem  ReferencedSubsystem=GasToAlpha
  XeGOut : Outport
  CxGas : Outport  Port=2
  wires:
  LiquidFlowRate/1 -> XeGOut/1, Add/3
  Subsystem/1 -> Add1/2, PreventDivideByZero/1
  LiquidVolume/1 -> LiquidFlowRate/2
  Add/1 -> PhaseMass/1
  Constant/1 -> Add1/1
  MixtureVolume/1 -> Divide/1, LiquidVolume/1
  Add1/1 -> LiquidVolume/2
  VolumeRate/1 -> LiquidFlowRate/1
  GasRef/1 -> Subsystem/1
  XeGIn/1 -> Add/1
  Gain2/1 -> Add/4
  PhaseMass/1 -> Gain2/1, MixtureVolume/1
  Interphase/1 -> Add/2
  PreventDivideByZero/1 -> Divide/2
  Constant1/1 -> PreventDivideByZero/2
  Divide/1 -> CxGas/1

== system MSDRPrimaryLoop_LoadFollow/Pump/PumpIdeal/XenonCalcPump/InterphaseTranfser ==
  note: This local to volume isn't strick. Either add an integral or reduce the length of the node if variation is large.
  CxSalt : Inport
  GasRef : Inport  Port=2
  CxGas : Inport  Port=3
  Constitutive : Subsystem
  MixtureVolume : Gain  Gain=PipeVolume
  Subsystem1 : Subsystem  ReferencedSubsystem=GasToAlpha
  Transfer Term : MATLAB Function  TreatAsAtomicUnit=on
  Ref : PMIOPort  Side=Left
  TranfserRate : Outport
  wires:
  Transfer Term/1(volRate) -> MixtureVolume/1
  MixtureVolume/1 -> TranfserRate/1
  Constitutive/3(k) -> Transfer Term/6(k)
  Constitutive/2(dsm) -> Transfer Term/5(dsm)
  GasRef/1 -> Subsystem1/1
  Subsystem1/1 -> Transfer Term/3(alpha)
  Constitutive/1(K) -> Transfer Term/4(K)
  CxSalt/1 -> Transfer Term/1(CxS)
  CxGas/1 -> Transfer Term/2(CxG)
  connections:
  Constitutive/LConn1 -- Ref/RConn1

== system MSDRPrimaryLoop_LoadFollow/Pump/PumpIdeal/XenonCalcPump/Salt ==
  XeLIn : Inport  PortDimensions=1
  IodineSNumberDensity : Inport  Port=2  PortDimensions=1
  T_f_ave : Inport  Port=3
  GasRef : Inport  Port=4  PortDimensions=1
  VolumeRate : Inport  Port=5
  Interphase : Inport  Port=6
  Add : Sum  Inputs=+++--  InputSameDT=on
  Decay : Gain  Gain=xeDecayConstant
  InPipeGeneration : Subsystem
      settings: PortSchema="{\"entries\":[{\"content\":{\"sides\":[{\"content\":{\"connectorIds\":[\"In1\"]},\"type\":\"ConnectorPlacement.EquallySpacedRectSide\",\"uuid\":\"cf58f9e2-4051-4ec0-bfd5-a375f3464f67\"},{\"content\":{\"connectorIds\":[\"Out1\"],\"side\":\"RIGHT\"},\"type\":\"ConnectorPlacement.EquallySpacedRectSide\",\"uuid\":\"cf475b22-0422-4ebc-b148-ab559744c6ba\"},{\"content\":{\"connectorIds\":[],\"side\":\"TOP\"},\"type\":\"ConnectorPlacement.EquallySpacedRectSide\",\"uuid\":\"15cc78ce-ee79-4f49-b098-b77c0b2a8ba1\"},{\"content\":{\"connectorIds\":[\"In2\"],\"side\":\"BOTTOM\"},\"type\":\"ConnectorPlacement.EquallySpacedRectSide\",\"uuid\":\"64f5be1f-19d6-4b5f-ac24-c41659a6a539\"}]},\"type\":\"ConnectorPlacement.EquallySpacedConnector\",\"uuid\":\"1fb1607a-ceed-4d70-a511-7b706be0d7ea\"}],\"packageUris\":[\"http://schema.mathworks.com/mf0/Connector/R2020b\"],\"version\":\"1.0\"}"
  LiquidFlowRate : Product
  LiquidVolume : Product  Inputs=*/
  MixtureVolume : Gain  Gain=1/PipeVolume
  PhaseMass : Integrator  LimitOutput=on  LowerSaturationLimit=0
  Subsystem1 : Subsystem
  XeLOut : Outport  PortDimensions=1
  CxSalt : Outport  Port=2
  wires:
  LiquidFlowRate/1 -> Add/5, XeLOut/1
  IodineSNumberDensity/1 -> InPipeGeneration/1(IodineSNumberDensity)
  LiquidVolume/1 -> CxSalt/1, LiquidFlowRate/2
  Add/1 -> PhaseMass/1
  MixtureVolume/1 -> LiquidVolume/1
  VolumeRate/1 -> LiquidFlowRate/1
  T_f_ave/1 -> InPipeGeneration/2(T_f_ave)
  PhaseMass/1 -> Decay/1, MixtureVolume/1
  GasRef/1 -> Subsystem1/1(Gas)
  Subsystem1/1(1-alpha) -> LiquidVolume/2
  InPipeGeneration/1("XenonGenerationRate, [kg/s]") -> Add/2
  XeLIn/1 -> Add/1
  Interphase/1 -> Add/3
  Decay/1 -> Add/4
